simulink model "LOSR"  (R2022a)
settings: Solver=FixedStepDiscrete  StartTime=0.0  StopTime=0.04  FixedStep=0.04  RelTol=1e-3
PreLoadFcn:
  | listing = dir;
  | if (contains([listing .name], 'AGR')) && (contains([listing .name], 'MAP'))
  |     addpath('./AGR', './MAP');
  |     addpath( genpath('./MAP') );
  | elseif (contains([listing .name], 'LOSR.slx'))
  |     addpath('../AGR', '../MAP');
  |     addpath( genpath('../MAP') );
  | else
  | 
  | end
  | 
  | load('BusStructureLOSR.mat');
InitFcn:
  | listing = dir;
  | if (contains([listing .name], 'AGR')) && (contains([listing .name], 'MAP'))
  |     addpath('./AGR', './MAP');
  |     addpath( genpath('./MAP') );
  | elseif (contains([listing .name], 'LOSR.slx'))
  |     addpath('../AGR', '../MAP');
  |     addpath( genpath('../MAP') );
  | else
  | 
  | end
  | 
  | load('BusStructureLOSR.mat');
StartFcn:
  | listing = dir;
  | if (contains([listing .name], 'AGR')) && (contains([listing .name], 'MAP'))
  |     addpath('./AGR', './MAP');
  |     addpath( genpath('./MAP') );
  | elseif (contains([listing .name], 'LOSR.slx'))
  |     addpath('../AGR', '../MAP');
  |     addpath( genpath('../MAP') );
  | else
  | 
  | end
  | 
  | load('BusStructureLOSR.mat');
undefined symbols (not defined in the file or in its folder): b2NED, dCNED, delECEF, isFeasible, llh, losECEF, LOSRDataTagWrap, LOSRDataValid, LOSRDirectionCosineX, LOSRDirectionCosineY, LOSRDirectionCosineZ, LOSRSelected, LOSRSelectedWraparound, LOSRTargetElevation, LOSRTargetLatitude, LOSRTargetLongitude, LOSRTargetRangeEast, LOSRTargetRangeNorth, LOSRTargetRangeVertical, ne, ned2ECEF, pECEF_ref, testLLH, testLLH2, testTerrainHeight
libraries: aerolibconvert2 x2
settings Model: Creator=ASCL  LastModifiedBy=ASCL
settings DataIOCC: SaveOutput=off  SignalLogging=off  DSMLogging=off  SaveTime=off  ReturnWorkspaceOutputs=off
settings OptimizationCC: BlockReduction=off  DefaultParameterBehavior=Inlined  UseDivisionForNetSlopeComputation=on  GainParamInheritBuiltInType=on  UseFloatMulNetSlope=on  ExpressionFolding=off  PassReuseOutputArgsAs=Individual arguments  ZeroExternalMemoryAtStartup=off  ZeroInternalMemoryAtStartup=off  EfficientFloat2IntCast=on  LifeSpan=inf  OptimizeBlockOrder=speed  DifferentSizesBufferReuse=on  EfficientTunableParamExpr=on
settings DebuggingCC: SignalInfNanChecking=warning  ReadBeforeWriteMsg=EnableAllAsWarning  WriteAfterWriteMsg=EnableAllAsError  WriteAfterReadMsg=EnableAllAsError  IntegerOverflowMsg=error  ParameterTunabilityLossMsg=error  UniqueDataStoreMsg=error  AssertControl=DisableAll  NonBusSignalsTreatedAsBus=error  SFInvalidInputDataAccessInChartInitDiag=error  SFTransitionOutsideNaturalParentDiag=error  SFUnreachableExecutionPathDiag=error  SFUndirectedBroadcastEventsDiag=error  IntegerSaturationMsg=error
settings HardwareCC: ProdBitPerPointer=32  ProdBitPerSizeT=32  ProdBitPerPtrDiffT=32  ProdLargestAtomicInteger=Long  ProdLargestAtomicFloat=Double  ProdEndianess=BigEndian  ProdWordSize=32  ProdLongLongMode=on  ProdHWDeviceType=Freescale->MPC83xx
settings ModelReferenceCC: ModelReferenceNumInstancesAllowed=Single
settings SFSimCC: SimCustomHeaderCode="#include \"MAP.h\""  SimUserSources=MAP.c  SimUserLibraries=WS2_32.LIB  CompileTimeRecursionLimit=0  EnableRuntimeRecursion=off  MATLABDynamicMemAlloc=off
settings RTWCC: SystemTargetFile=ert.tlc  TemplateMakefile=ert_default_tmf  GenerateReport=on  RTWUseSimCustomCode=on  CustomHeaderCode="#include \"MAP.h\""  CustomSource=MAP.c  CustomLibrary=WS2_32.LIB  BuildConfiguration=Faster Runs  IncludeHyperlinkInReport=on  LaunchReport=on  GenerateTraceInfo=on  GenerateTraceReport=on  GenerateTraceReportSl=on  GenerateTraceReportSf=on  GenerateTraceReportEml=on  GenerateCodeMetricsReport=on
settings CodeAppCC: ForceParamTrailComments=on  IgnoreCustomStorageClasses=off  OperatorAnnotations=on  SimulinkDataObjDesc=on  SFDataObjDesc=on  MATLABFcnDesc=on  InsertBlockDesc=on  StateflowObjectComments=on  MATLABSourceComments=on  EnableCustomComments=on  InlinedPrmAccess=Macros  ReqsInCode=on
settings ERTTargetCC: TargetLangStandard=C99 (ISO)  UtilityFuncGeneration=Shared location  GenerateSampleERTMain=on  IncludeMdlTerminateFcn=off  CombineSignalStateStructs=on  SuppressErrorStatus=on  SupportAbsoluteTime=off  SupportNonFinite=off  SupportComplex=off  SupportVariableSizeSignals=on  ParenthesesLevel=Standards  CastingMode=Standards  GenerateSharedConstants=off  InlinedParameterPlacement=NonHierarchical  ERTCustomFileTemplate=example_file_process.tlc  RateTransitionBlockCode=Function  PreserveIfCondition=on  ConvertIfToSwitch=off  EnableSignedLeftShifts=off  EnableSignedRightShifts=off

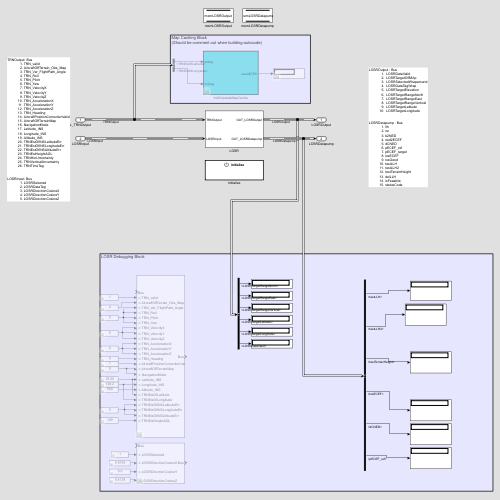
[thumbnail: Simulink's stored preview of the top-level diagram]
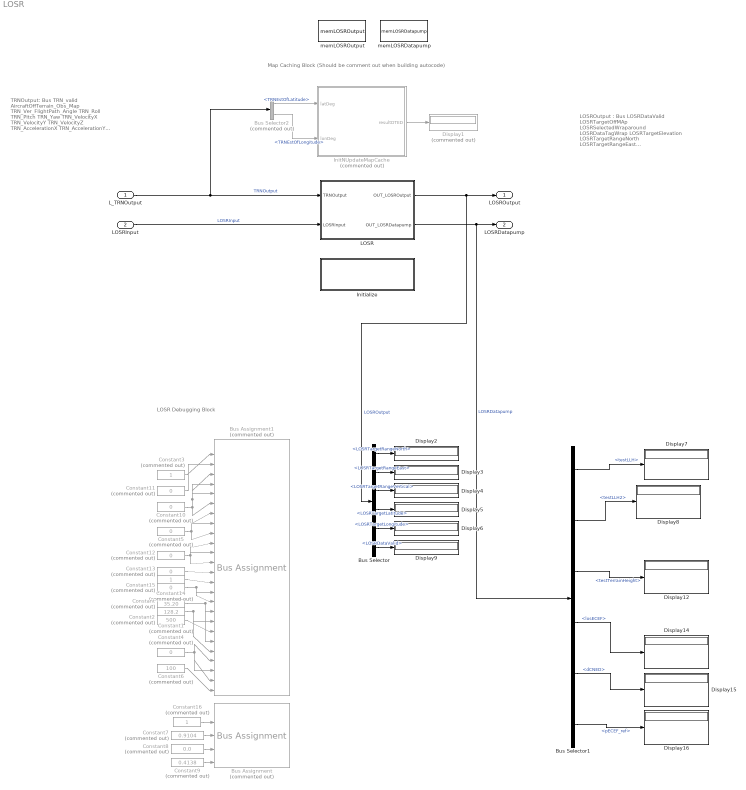
== system LOSR ==
  note: LOSR Debugging Block
  note: LOSROutput : Bus
      | LOSRDataValid
      | LOSRTargetOffMAp
      | LOSRSelectedWraparound
      | LOSRDataTagWrap
      | LOSRTargetElevation
      | LOSRTargetRangeNorth
      | LOSRTargetRangeEast
      | LOSRTargetRangeVertical
      | LOSRTargetLatitude
      | LOSRTargetLongitude
      |
      | LOSRDatapump : Bus
      | llh
      | ne
      | b2NED
      | ned2ECEF
      | dCNED
      | pECEF_ref
      | pECEF_target
      | losECEF
      | losGeod
      | testLLH
      | testLLH2
      | testTerrainHeight
      | delLLH
      | isFeasbile
      | statusCode
  note: TRNOutput: Bus
      | TRN_valid
      | AircraftOffTerrain_Obs_Map
      | TRN_Ver_FlightPath_Angle
      | TRN_Roll
      | TRN_Pitch
      | TRN_Yaw
      | TRN_VelocityX
      | TRN_VelocityY
      | TRN_VelocityZ
      | TRN_AccelerationX
      | TRN_AccelerationY
      | TRN_AccelerationZ
      | TRN_Heading
      | AircraftPositionCorrectionValid
      | AircraftOffTerrainMap
      | NavigationMode
      | Latitude_INS
      | Longitude_INS
      | Altitude_INS
      | TRNEstOfINSLatitudeErr
      | TRNEstOfINSLongitudeErr
      | TRNEstOfINSAltitudeErr
      | TRNEstHeightAGL
      | TRNHorUncertainty
      | TRNVerticalUncertainty
      | TRNTimeTag
      |
      | LOSRInput: Bus
      | LOSRSelected
      | LOSRDataTag
      | LOSRDirectionCosineX
      | LOSRDirectionCosineY
      | LOSRDirectionCosineZ
  note: Map Caching Block
      | (Should be comment out when building autocode)
  L_TRNOutput : Inport  OutDataTypeStr=Bus: TRNOutput  Interpolate=off  BusOutputAsStruct=on
  LOSRInput : Inport  Port=2  OutDataTypeStr=Bus: LOSRInput  Interpolate=off  BusOutputAsStruct=on
  Bus Assignment : BusAssignment  Commented=on  AssignedSignals=LOSRSelected,LOSRDirectionCosineX,LOSRDirectionCosineY,LOSRDirectionCosineZ
  Bus Assignment1 : BusAssignment  Commented=on  AssignedSignals=TRN_valid,AircraftOffTerrain_Obs_Map,TRN_Ver_FlightPath_Angle,TRN_Roll,TRN_Pitch,TRN_Yaw,TRN_VelocityX,TRN_VelocityY,TRN_VelocityZ,TRN_AccelerationX,TRN_AccelerationY,TRN_AccelerationZ,TRN_Heading,AircraftPositionCorrectionValid,AircraftOffTerrainMap,NavigationMode,Latitude_INS,Longitude_INS,Altitude_INS,TRNEstOfLatitude,TRNEstOfLongitude,TRNEstOfINSLatitudeErr,TRNEstOfINSLongitudeErr,TRNEstOfINSAltitudeErr,TRNEstHeightAGL
  Bus Selector : BusSelector  OutputSignals=LOSRTargetRangeNorth,LOSRTargetRangeEast,LOSRTargetRangeVertical,LOSRTargetLatitude,LOSRTargetLongitude,LOSRDataValid
  Bus Selector1 : BusSelector  OutputSignals=testLLH,testLLH2,testTerrainHeight,losECEF,dCNED,pECEF_ref
  Bus Selector2 : BusSelector  Commented=on  OutputSignals=TRNEstOfLatitude,TRNEstOfLongitude
  Constant : Constant  Commented=on  Value=35.20
  Constant1 : Constant  Commented=on  Value=128.2
  Constant{4..5,10,12..13} (5 alike) : Constant  Commented=on  Value=0
  Constant11 : Constant  Commented=on  Value=0  OutDataTypeStr=boolean
  Constant14 : Constant  Commented=on  OutDataTypeStr=boolean
  Constant15 : Constant  Commented=on  Value=0  OutDataTypeStr=boolean
  Constant16 : Constant  Commented=on  OutDataTypeStr=boolean
  Constant2 : Constant  Commented=on  Value=500
  Constant3 : Constant  Commented=on  OutDataTypeStr=boolean
  Constant6 : Constant  Commented=on  Value=100  OutDataTypeStr=uint16
  Constant7 : Constant  Commented=on  Value=0.9104
  Constant8 : Constant  Commented=on  Value=0.0
  Constant9 : Constant  Commented=on  Value=0.4138
  Display1 : Display  Commented=on
  Display{2..9,12,14..16} (12 alike) : Display
  InitNUpdateMapCache : Subsystem  Commented=on  TreatAsAtomicUnit=on
  Initialize : Subsystem  TreatAsAtomicUnit=on
  LOSR : Subsystem
      mask init:
      | % latGPS = double(0);
      | % lonGPS = double(0);
      | % altGPS = double(0);
      | % velEGPS = double(0);
      | % velNGPS = double(0);
      | % velUGPS = double(0);
      | % notValidGPS = boolean(0);
      | % notAvaildINS = boolean(0);
      | % velUINS = double(0);
      | % velVINS = double(0);
      | % velWINS = double(0);
      | % rollINS = double(0);
      | % pitchINS = double(0);
      | % hgdINS = double(0);
      | % accXINS = double(0);
      | % accYINS = double(0);
      | % accZINS = double(0);
      | % activated = boolean(0);
      | % reactionT = uint16(0);
      | % pullUpG = uint16(0);
      | % rollRate = uint16(0);
      | % gOnsetRate = uint16(0);
      | % maxGamma = uint16(0);
      | % setWarnH = double(0);
      | % obsWarningTime = uint16(1);
      | % wiresWarningTime = uint16(1);
      | % latErrOfINS = double(0);
      | % lonErrOfINS = double(0);
      | % altErrorofINS = uint16(0);
      | % heightEstOfTRN = uint16(0);
      | % horUncertaintyOfTRN = double(0);
      | % verUncertaintyOfTRN = double(0);
  memLOSRDatapump : DataStoreMemory  DataStoreName=memLOSRDatapump  ReadBeforeWriteMsg=warning  WriteAfterWriteMsg=warning  WriteAfterReadMsg=warning  VectorParams1D=off  ShowAdditionalParam=off  OutDataTypeStr=Bus: LOSRDatapump
  memLOSROutput : DataStoreMemory  DataStoreName=memLOSROutput  ReadBeforeWriteMsg=warning  WriteAfterWriteMsg=warning  WriteAfterReadMsg=warning  VectorParams1D=off  ShowAdditionalParam=off  OutDataTypeStr=Bus: LOSROutput
  LOSROutput : Outport  OutDataTypeStr=Bus: LOSROutput  VectorParamsAs1DForOutWhenUnconnected=off  BusOutputAsStruct=on
  LOSRDatapump : Outport  Port=2  OutDataTypeStr=Bus: LOSRDatapump  VectorParamsAs1DForOutWhenUnconnected=off  BusOutputAsStruct=on
  wires:
  Constant11/1 -> Bus Assignment1/3
  Constant2/1 -> Bus Assignment1/20
  L_TRNOutput/1 -> Bus Selector2/1, LOSR/1(TRNOutput)  "TRNOutput"
  Constant16/1 -> Bus Assignment/2
  Constant10/1 -> Bus Assignment1/7, Bus Assignment1/4, Bus Assignment1/5, Bus Assignment1/6
  Constant6/1 -> Bus Assignment1/26
  Bus Selector2/2 -> InitNUpdateMapCache/2(lonDeg)  "<TRNEstOfLongitude>"
  Bus Selector/5 -> Display6/1  "<LOSRTargetLongitude>"
  LOSR/2(OUT_LOSRDatapump) -> Bus Selector1/1, LOSRDatapump/1  "LOSRDatapump"
  LOSRInput/1 -> LOSR/2(LOSRInput)  "LOSRInput"
  Constant9/1 -> Bus Assignment/5
  Constant7/1 -> Bus Assignment/3
  Constant1/1 -> Bus Assignment1/22, Bus Assignment1/19
  Bus Selector/2 -> Display3/1  "<LOSRTargetRangeEast>"
  Bus Selector1/2 -> Display8/1  "<testLLH2>"
  Bus Selector1/5 -> Display15/1  "<dCNED>"
  Constant13/1 -> Bus Assignment1/14
  Constant15/1 -> Bus Assignment1/17, Bus Assignment1/16
  Bus Selector/6 -> Display9/1  "<LOSRDataValid>"
  LOSR/1(OUT_LOSROutput) -> Bus Selector/1, LOSROutput/1  "LOSROutput"
  Bus Selector2/1 -> InitNUpdateMapCache/1(latDeg)  "<TRNEstOfLatitude>"
  Constant14/1 -> Bus Assignment1/15
  Bus Selector1/1 -> Display7/1  "<testLLH>"
  Constant12/1 -> Bus Assignment1/13, Bus Assignment1/11, Bus Assignment1/12
  Bus Selector1/6 -> Display16/1  "<pECEF_ref>"
  Constant3/1 -> Bus Assignment1/2
  Constant5/1 -> Bus Assignment1/10, Bus Assignment1/8, Bus Assignment1/9
  Constant4/1 -> Bus Assignment1/23, Bus Assignment1/25, Bus Assignment1/24
  Constant/1 -> Bus Assignment1/21, Bus Assignment1/18
  Bus Selector/4 -> Display5/1  "<LOSRTargetLatitude>"
  Bus Selector/3 -> Display4/1  "<LOSRTargetRangeVertical>"
  Bus Selector/1 -> Display2/1  "<LOSRTargetRangeNorth>"
  Bus Selector1/4 -> Display14/1  "<losECEF>"
  Constant8/1 -> Bus Assignment/4
  Bus Selector1/3 -> Display12/1  "<testTerrainHeight>"
  InitNUpdateMapCache/1(resultDTED) -> Display1/1

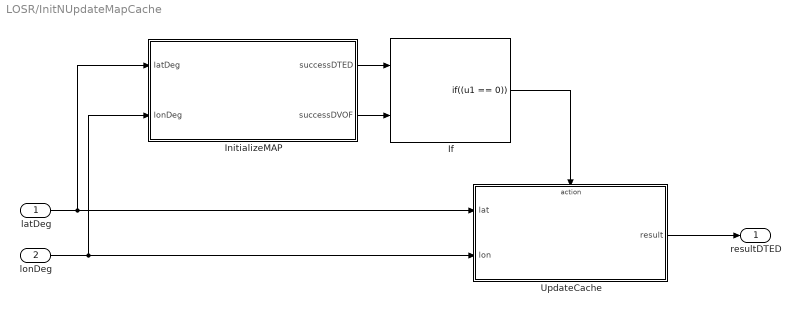
== system LOSR/InitNUpdateMapCache ==
  latDeg : Inport  OutDataTypeStr=double
  lonDeg : Inport  Port=2  OutDataTypeStr=double
  If : If  NumInputs=2  IfExpression=(u1 == 0)  ShowElse=off
  InitializeMAP : MATLAB Function  TreatAsAtomicUnit=on
  UpdateCache : Subsystem  TreatAsAtomicUnit=on
  resultDTED : Outport  VectorParamsAs1DForOutWhenUnconnected=off
  wires:
  lonDeg/1 -> InitializeMAP/2(lonDeg), UpdateCache/2(lon)
  UpdateCache/1(result) -> resultDTED/1
  InitializeMAP/1(successDTED) -> If/1
  latDeg/1 -> InitializeMAP/1(latDeg), UpdateCache/1(lat)
  InitializeMAP/2(successDVOF) -> If/2
  If/1 -> UpdateCache/Action

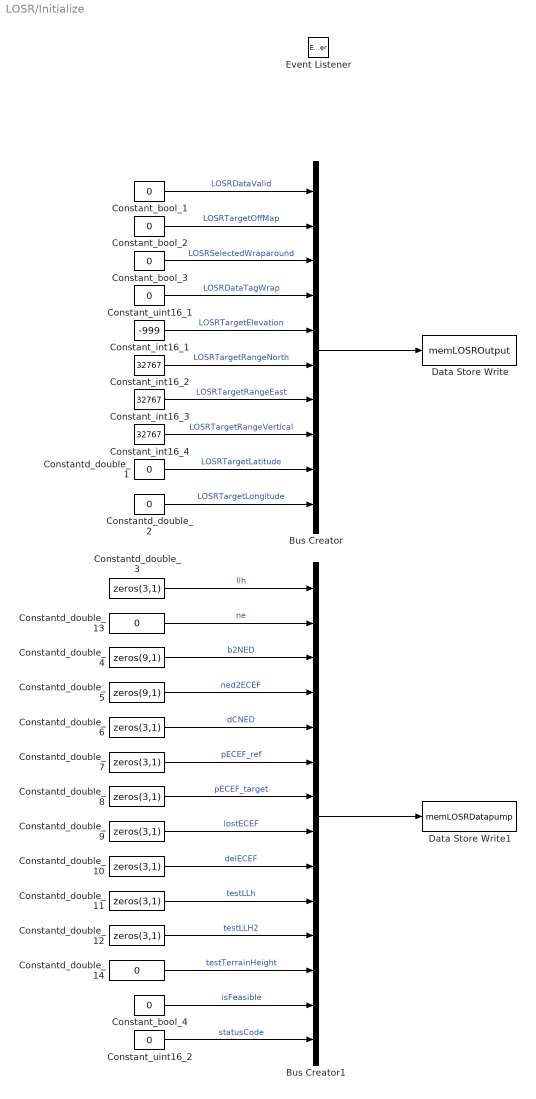
== system LOSR/Initialize ==
  Bus Creator : BusCreator  Inputs=10  OutDataTypeStr=Bus: LOSROutput  NonVirtualBus=on
      settings: InheritFromInputs=off
  Bus Creator1 : BusCreator  Inputs=14  OutDataTypeStr=Bus: LOSRDatapump  NonVirtualBus=on
      settings: InheritFromInputs=off
  Constant_bool_{1..4} (4 alike) : Constant  Value=0  OutDataTypeStr=boolean
  Constant_int16_1 : Constant  Value=-999  OutDataTypeStr=int16
  Constant_int16_2 : Constant  Value=32767  OutDataTypeStr=int16
  Constant_int16_3 : Constant  Value=32767  OutDataTypeStr=int16
  Constant_int16_4 : Constant  Value=32767  OutDataTypeStr=int16
  Constant_uint16_1 : Constant  Value=0  OutDataTypeStr=uint16
  Constant_uint16_2 : Constant  Value=0  OutDataTypeStr=uint16
  Constantd_double_{1..2,13..14} (4 alike) : Constant  Value=0  OutDataTypeStr=double
  Constantd_double_{3,6..12} (8 alike) : Constant  Value=zeros(3,1)  OutDataTypeStr=double
  Constantd_double_4 : Constant  Value=zeros(9,1)  OutDataTypeStr=double
  Constantd_double_5 : Constant  Value=zeros(9,1)  OutDataTypeStr=double
  Data Store Write : DataStoreWrite  DataStoreName=memLOSROutput  IndexOptions=Index vector (dialog)  Indices=1  OutputSizes=1
  Data Store Write1 : DataStoreWrite  DataStoreName=memLOSRDatapump  IndexOptions=Index vector (dialog)  Indices=1  OutputSizes=1
  Event Listener : EventListener  DisableCoverage=on  EventName=reset
  wires:
  Constant_uint16_1/1 -> Bus Creator/4  "LOSRDataTagWrap"
  Constant_bool_1/1 -> Bus Creator/1  "LOSRDataValid"
  Constant_bool_2/1 -> Bus Creator/2  "LOSRTargetOffMap"
  Constant_bool_3/1 -> Bus Creator/3  "LOSRSelectedWraparound"
  Constant_int16_1/1 -> Bus Creator/5  "LOSRTargetElevation"
  Constant_int16_2/1 -> Bus Creator/6  "LOSRTargetRangeNorth"
  Constant_int16_3/1 -> Bus Creator/7  "LOSRTargetRangeEast"
  Constant_int16_4/1 -> Bus Creator/8  "LOSRTargetRangeVertical"
  Constantd_double_1/1 -> Bus Creator/9  "LOSRTargetLatitude"
  Constantd_double_2/1 -> Bus Creator/10  "LOSRTargetLongitude"
  Bus Creator/1 -> Data Store Write/1
  Bus Creator1/1 -> Data Store Write1/1
  Constantd_double_3/1 -> Bus Creator1/1  "llh"
  Constantd_double_4/1 -> Bus Creator1/3  "b2NED"
  Constantd_double_5/1 -> Bus Creator1/4  "ned2ECEF"
  Constantd_double_8/1 -> Bus Creator1/7  "pECEF_target"
  Constantd_double_7/1 -> Bus Creator1/6  "pECEF_ref"
  Constantd_double_6/1 -> Bus Creator1/5  "dCNED"
  Constantd_double_9/1 -> Bus Creator1/8  "lostECEF"
  Constantd_double_10/1 -> Bus Creator1/9  "delECEF"
  Constantd_double_11/1 -> Bus Creator1/10  "testLLh"
  Constantd_double_12/1 -> Bus Creator1/11  "testLLH2"
  Constantd_double_13/1 -> Bus Creator1/2  "ne"
  Constantd_double_14/1 -> Bus Creator1/12  "testTerrainHeight"
  Constant_bool_4/1 -> Bus Creator1/13  "isFeasible"
  Constant_uint16_2/1 -> Bus Creator1/14  "statusCode"

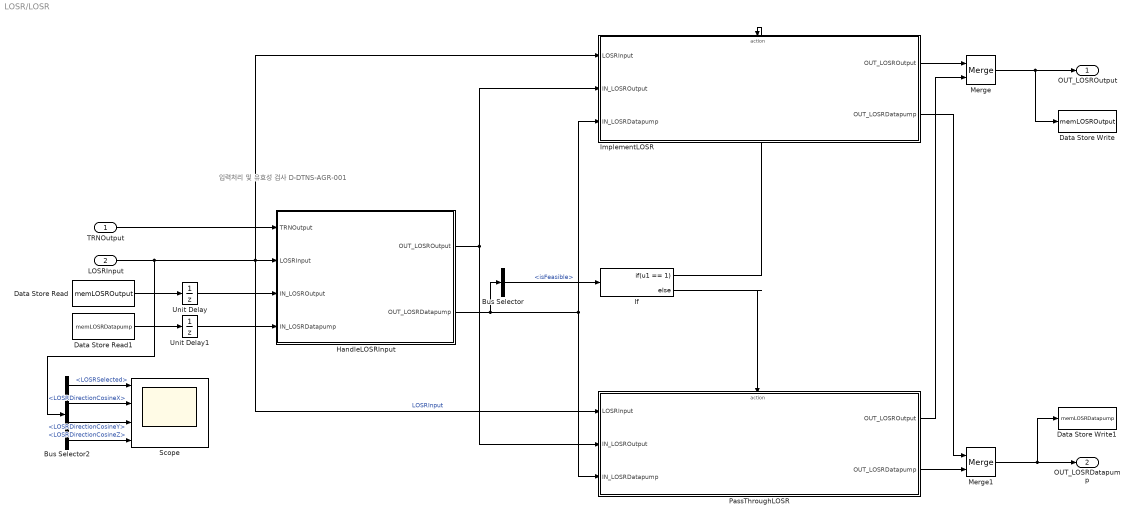
== system LOSR/LOSR ==
  note: 입력처리 및 유효성 검사 D-DTNS-AGR-001
  TRNOutput : Inport  OutDataTypeStr=Bus: TRNOutput
  LOSRInput : Inport  Port=2  OutDataTypeStr=Bus: LOSRInput
  Bus Selector : BusSelector  OutputSignals=isFeasible
  Bus Selector2 : BusSelector  OutputSignals=LOSRSelected,LOSRDirectionCosineX,LOSRDirectionCosineY,LOSRDirectionCosineZ
  Data Store Read : DataStoreRead  DataStoreName=memLOSROutput  IndexOptions=Index vector (dialog)  Indices=1  OutputSizes=1
  Data Store Read1 : DataStoreRead  DataStoreName=memLOSRDatapump  IndexOptions=Index vector (dialog)  Indices=1  OutputSizes=1
  Data Store Write : DataStoreWrite  DataStoreName=memLOSROutput  IndexOptions=Index vector (dialog)  Indices=1  OutputSizes=1
  Data Store Write1 : DataStoreWrite  DataStoreName=memLOSRDatapump  IndexOptions=Index vector (dialog)  Indices=1  OutputSizes=1
  HandleLOSRInput : Subsystem  TreatAsAtomicUnit=on
      settings: RTWSystemCode=Nonreusable function  RTWFcnNameOpts=Use subsystem name
  If : If  IfExpression=u1 == 1
  ImplementLOSR : Subsystem  TreatAsAtomicUnit=on
      settings: RTWSystemCode=Nonreusable function  RTWFcnNameOpts=Use subsystem name
  Merge : Merge
  Merge1 : Merge
  PassThroughLOSR : Subsystem  TreatAsAtomicUnit=on
      settings: RTWSystemCode=Nonreusable function  RTWFcnNameOpts=Use subsystem name
  Scope : Scope  NumInputPorts=4
  Unit Delay : UnitDelay  SampleTime=-1  HasFrameUpgradeWarning=on
  Unit Delay1 : UnitDelay  SampleTime=-1  HasFrameUpgradeWarning=on
  OUT_LOSROutput : Outport  OutDataTypeStr=Bus: LOSROutput  VectorParamsAs1DForOutWhenUnconnected=off
  OUT_LOSRDatapump : Outport  Port=2  OutDataTypeStr=Bus: LOSRDatapump  VectorParamsAs1DForOutWhenUnconnected=off
  wires:
  LOSRInput/1 -> Bus Selector2/1, ImplementLOSR/1(LOSRInput), PassThroughLOSR/1(LOSRInput), HandleLOSRInput/2(LOSRInput)  "LOSRInput"
  HandleLOSRInput/1(OUT_LOSROutput) -> PassThroughLOSR/2(IN_LOSROutput), ImplementLOSR/2(IN_LOSROutput)
  Bus Selector/1 -> If/1  "<isFeasible>"
  If/1 -> ImplementLOSR/Action
  HandleLOSRInput/2(OUT_LOSRDatapump) -> Bus Selector/1, ImplementLOSR/3(IN_LOSRDatapump), PassThroughLOSR/3(IN_LOSRDatapump)
  ImplementLOSR/1(OUT_LOSROutput) -> Merge/1
  PassThroughLOSR/2(OUT_LOSRDatapump) -> Merge1/2
  ImplementLOSR/2(OUT_LOSRDatapump) -> Merge1/1
  PassThroughLOSR/1(OUT_LOSROutput) -> Merge/2
  Merge/1 -> Data Store Write/1, OUT_LOSROutput/1
  Merge1/1 -> Data Store Write1/1, OUT_LOSRDatapump/1
  If/2 -> PassThroughLOSR/Action
  TRNOutput/1 -> HandleLOSRInput/1(TRNOutput)
  Data Store Read/1 -> Unit Delay/1
  Data Store Read1/1 -> Unit Delay1/1
  Unit Delay/1 -> HandleLOSRInput/3(IN_LOSROutput)
  Unit Delay1/1 -> HandleLOSRInput/4(IN_LOSRDatapump)
  Bus Selector2/1 -> Scope/1  "<LOSRSelected>"
  Bus Selector2/2 -> Scope/2  "<LOSRDirectionCosineX>"
  Bus Selector2/3 -> Scope/3  "<LOSRDirectionCosineY>"
  Bus Selector2/4 -> Scope/4  "<LOSRDirectionCosineZ>"

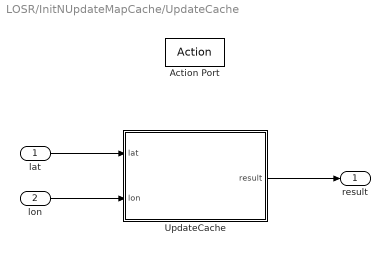
== system LOSR/InitNUpdateMapCache/UpdateCache ==
  lat : Inport
  lon : Inport  Port=2
  Action Port : ActionPort
  UpdateCache : MATLAB Function  TreatAsAtomicUnit=on
  result : Outport  VectorParamsAs1DForOutWhenUnconnected=off
  wires:
  UpdateCache/1(result) -> result/1
  lat/1 -> UpdateCache/1(lat)
  lon/1 -> UpdateCache/2(lon)

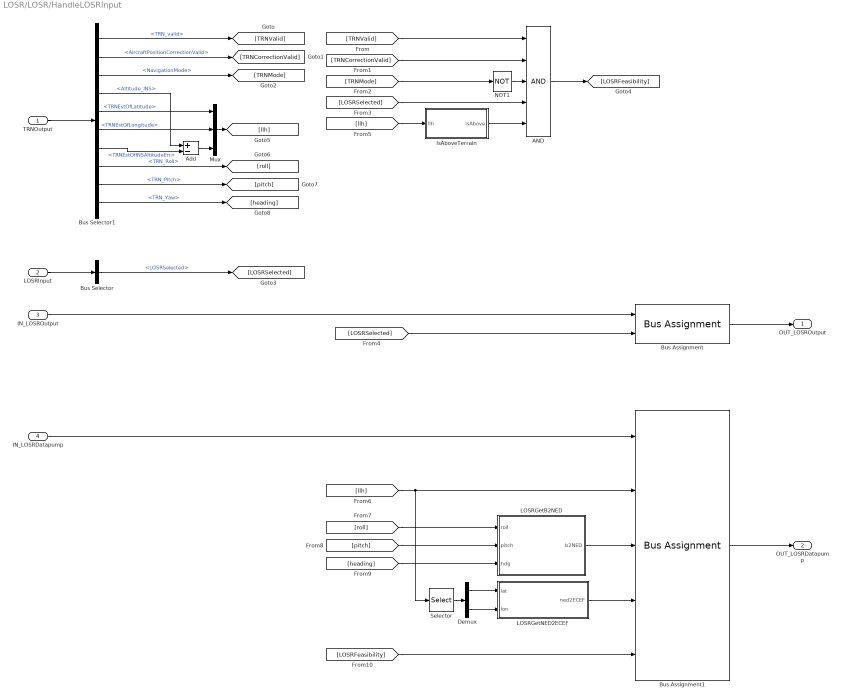
== system LOSR/LOSR/HandleLOSRInput ==
  TRNOutput : Inport  OutDataTypeStr=Bus: TRNOutput
  LOSRInput : Inport  Port=2  OutDataTypeStr=Bus: LOSRInput
  IN_LOSROutput : Inport  Port=3  OutDataTypeStr=Bus: LOSROutput
  IN_LOSRDatapump : Inport  Port=4  OutDataTypeStr=Bus: LOSRDatapump
  AND : Logic  Inputs=5  AllPortsSameDT=off  OutDataTypeStr=boolean
  Add : Sum  Inputs=+-
  Bus Assignment : BusAssignment  AssignedSignals=LOSRSelectedWraparound
  Bus Assignment1 : BusAssignment  AssignedSignals=llh,b2NED,ned2ECEF,isFeasible
  Bus Selector : BusSelector  OutputSignals=LOSRSelected
  Bus Selector1 : BusSelector  OutputSignals=TRN_valid,AircraftPositionCorrectionValid,NavigationMode,Altitude_INS,TRNEstOfLatitude,TRNEstOfLongitude,TRNEstOfINSAltitudeErr,TRN_Roll,TRN_Pitch,TRN_Yaw
  Demux : Demux  Outputs=2
  IsAboveTerrain : MATLAB Function  TreatAsAtomicUnit=on
  LOSRGetB2NED : MATLAB Function  TreatAsAtomicUnit=on
  LOSRGetNED2ECEF : MATLAB Function  TreatAsAtomicUnit=on
  Mux : Mux  Inputs=3
  NOT1 : Logic  Operator=NOT  IconShape=distinctive  AllPortsSameDT=off  OutDataTypeStr=boolean
  Selector : Selector  InputPortWidth=3  IndexOptions=Index vector (dialog)  Indices=[1 2]  OutputSizes=1
  OUT_LOSROutput : Outport  OutDataTypeStr=Bus: LOSROutput  VectorParamsAs1DForOutWhenUnconnected=off
  OUT_LOSRDatapump : Outport  Port=2  OutDataTypeStr=Bus: LOSRDatapump  VectorParamsAs1DForOutWhenUnconnected=off
  wires:
  IN_LOSRDatapump/1 -> Bus Assignment1/1
  IN_LOSROutput/1 -> Bus Assignment/1
  TRNOutput/1 -> Bus Selector1/1
  Bus Selector1/1 -> [TRNValid]  "<TRN_valid>"
  Bus Selector1/2 -> [TRNCorrectionValid]  "<AircraftPositionCorrectionValid>"
  Bus Selector1/3 -> [TRNMode]  "<NavigationMode>"
  LOSRInput/1 -> Bus Selector/1
  Bus Selector/1 -> [LOSRSelected]  "<LOSRSelected>"
  [TRNValid] -> AND/1
  [TRNCorrectionValid] -> AND/2
  [TRNMode] -> NOT1/1
  [LOSRSelected] -> AND/4
  AND/1 -> [LOSRFeasibility]
  Bus Assignment1/1 -> OUT_LOSRDatapump/1
  LOSRGetNED2ECEF/1(ned2ECEF) -> Bus Assignment1/4
  LOSRGetB2NED/1(b2NED) -> Bus Assignment1/3
  Bus Selector1/4 -> Add/1  "<Altitude_INS>"
  Bus Selector1/5 -> Mux/1  "<TRNEstOfLatitude>"
  Bus Selector1/6 -> Mux/2  "<TRNEstOfLongitude>"
  Add/1 -> Mux/3
  Bus Selector1/7 -> Add/2  "<TRNEstOfINSAltitudeErr>"
  Mux/1 -> [llh]
  Bus Selector1/10 -> [heading]  "<TRN_Yaw>"
  Bus Selector1/9 -> [pitch]  "<TRN_Pitch>"
  Bus Selector1/8 -> [roll]  "<TRN_Roll>"
  [llh] -> Selector/1, Bus Assignment1/2
  Selector/1 -> Demux/1
  Demux/2 -> LOSRGetNED2ECEF/2(lon)
  Demux/1 -> LOSRGetNED2ECEF/1(lat)
  [roll] -> LOSRGetB2NED/1(roll)
  [pitch] -> LOSRGetB2NED/2(pitch)
  [heading] -> LOSRGetB2NED/3(hdg)
  NOT1/1 -> AND/3
  [LOSRFeasibility] -> Bus Assignment1/5
  Bus Assignment/1 -> OUT_LOSROutput/1
  [LOSRSelected] -> Bus Assignment/2
  [llh] -> IsAboveTerrain/1(llh)
  IsAboveTerrain/1(isAbove) -> AND/5

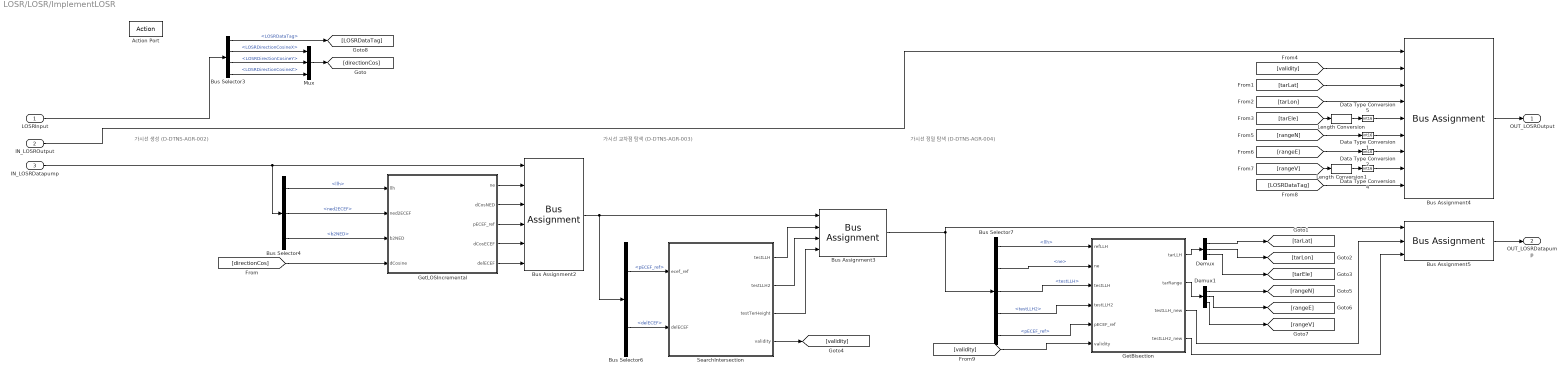
== system LOSR/LOSR/ImplementLOSR ==
  note: 가시선 생성 (D-DTNS-AGR-002)
  note: 가시선 교차점 탐색 (D-DTNS-AGR-003)
  note: 가시선 정밀 탐색 (D-DTNS-AGR-004)
  LOSRInput : Inport  OutDataTypeStr=Bus: LOSRInput
  IN_LOSROutput : Inport  Port=2  OutDataTypeStr=Bus: LOSROutput
  IN_LOSRDatapump : Inport  Port=3  OutDataTypeStr=Bus: LOSRDatapump
  Action Port : ActionPort  ActionPortLabel=if(u1 == 1)
  Bus Assignment2 : BusAssignment  AssignedSignals=ne,dCNED,pECEF_ref,losECEF,delECEF
  Bus Assignment3 : BusAssignment  AssignedSignals=testLLH,testLLH2,testTerrainHeight
  Bus Assignment4 : BusAssignment  AssignedSignals=LOSRDataValid,LOSRTargetLatitude,LOSRTargetLongitude,LOSRTargetElevation,LOSRTargetRangeNorth,LOSRTargetRangeEast,LOSRTargetRangeVertical,LOSRDataTagWrap
  Bus Assignment5 : BusAssignment  AssignedSignals=testLLH,testLLH2
  Bus Selector3 : BusSelector  OutputSignals=LOSRDataTag,LOSRDirectionCosineX,LOSRDirectionCosineY,LOSRDirectionCosineZ
  Bus Selector4 : BusSelector  OutputSignals=llh,ned2ECEF,b2NED
  Bus Selector6 : BusSelector  OutputSignals=pECEF_ref,delECEF
  Bus Selector7 : BusSelector  OutputSignals=llh,ne,testLLH,testLLH2,pECEF_ref
  Data Type Conversion{1..2,4..5} (4 alike) : DataTypeConversion  OutDataTypeStr=int16  RndMeth=Floor
  Demux : Demux  Outputs=3
  Demux1 : Demux  Outputs=3
  GetBisection : MATLAB Function  TreatAsAtomicUnit=on
      settings: RTWSystemCode=Nonreusable function  RTWFcnNameOpts=Use subsystem name
  GetLOSIncremental : MATLAB Function  TreatAsAtomicUnit=on
      settings: RTWSystemCode=Nonreusable function  RTWFcnNameOpts=Use subsystem name
  Length Conversion : aerolibconvert2/Length Conversion  IU=m  OU=ft
  Length Conversion1 : aerolibconvert2/Length Conversion  IU=m  OU=ft
  Mux : Mux  Inputs=3
  SearchIntersection : MATLAB Function  TreatAsAtomicUnit=on
      settings: RTWSystemCode=Nonreusable function  RTWFcnNameOpts=Use subsystem name
  OUT_LOSROutput : Outport  OutDataTypeStr=Bus: LOSROutput  VectorParamsAs1DForOutWhenUnconnected=off
  OUT_LOSRDatapump : Outport  Port=2  OutDataTypeStr=Bus: LOSRDatapump  VectorParamsAs1DForOutWhenUnconnected=off
  wires:
  Bus Assignment3/1 -> Bus Selector7/1, Bus Assignment5/1
  SearchIntersection/4(validity) -> [validity]
  [tarLat] -> Bus Assignment4/3
  SearchIntersection/1(testLLH) -> Bus Assignment3/2
  [rangeV] -> Length Conversion1/1
  [directionCos] -> GetLOSIncremental/4(dCosine)
  [tarEle] -> Length Conversion/1
  Bus Selector4/3 -> GetLOSIncremental/3(b2NED)  "<b2NED>"
  Bus Assignment2/1 -> Bus Selector6/1, Bus Assignment3/1
  [tarLon] -> Bus Assignment4/4
  Bus Selector3/3 -> Mux/2  "<LOSRDirectionCosineY>"
  Bus Selector3/2 -> Mux/1  "<LOSRDirectionCosineX>"
  IN_LOSRDatapump/1 -> Bus Selector4/1, Bus Assignment2/1
  Bus Selector4/1 -> GetLOSIncremental/1(llh)  "<llh>"
  Bus Selector3/1 -> [LOSRDataTag]  "<LOSRDataTag>"
  Bus Selector4/2 -> GetLOSIncremental/2(ned2ECEF)  "<ned2ECEF>"
  IN_LOSROutput/1 -> Bus Assignment4/1
  [rangeN] -> Data Type Conversion1/1
  Demux1/2 -> [rangeE]
  Demux1/1 -> [rangeN]
  Mux/1 -> [directionCos]
  [rangeE] -> Data Type Conversion2/1
  Demux/3 -> [tarEle]
  SearchIntersection/3(testTerHeight) -> Bus Assignment3/4
  Demux1/3 -> [rangeV]
  [validity] -> Bus Assignment4/2
  LOSRInput/1 -> Bus Selector3/1
  Bus Assignment4/1 -> OUT_LOSROutput/1
  Bus Assignment5/1 -> OUT_LOSRDatapump/1
  Bus Selector3/4 -> Mux/3  "<LOSRDirectionCosineZ>"
  [LOSRDataTag] -> Bus Assignment4/9
  GetLOSIncremental/5(delECEF) -> Bus Assignment2/6
  GetLOSIncremental/1(ne) -> Bus Assignment2/2
  GetLOSIncremental/2(dCosNED) -> Bus Assignment2/3
  GetLOSIncremental/3(pECEF_ref) -> Bus Assignment2/4
  GetLOSIncremental/4(dCosECEF) -> Bus Assignment2/5
  Bus Selector6/1 -> SearchIntersection/1(ecef_ref)  "<pECEF_ref>"
  Bus Selector6/2 -> SearchIntersection/2(delECEF)  "<delECEF>"
  SearchIntersection/2(testLLH2) -> Bus Assignment3/3
  Bus Selector7/1 -> GetBisection/1(refLLH)  "<llh>"
  Bus Selector7/2 -> GetBisection/2(ne)  "<ne>"
  Bus Selector7/3 -> GetBisection/3(testLLH)  "<testLLH>"
  Bus Selector7/4 -> GetBisection/4(testLLH2)  "<testLLH2>"
  Bus Selector7/5 -> GetBisection/5(pECEF_ref)  "<pECEF_ref>"
  GetBisection/1(tarLLH) -> Demux/1
  Demux/1 -> [tarLat]
  Demux/2 -> [tarLon]
  GetBisection/2(tarRange) -> Demux1/1
  GetBisection/4(testLLH2_new) -> Bus Assignment5/3
  GetBisection/3(testLLH_new) -> Bus Assignment5/2
  [validity] -> GetBisection/6(validity)
  Length Conversion/1 -> Data Type Conversion5/1
  Data Type Conversion4/1 -> Bus Assignment4/8
  Data Type Conversion5/1 -> Bus Assignment4/5
  Length Conversion1/1 -> Data Type Conversion4/1
  Data Type Conversion1/1 -> Bus Assignment4/6
  Data Type Conversion2/1 -> Bus Assignment4/7

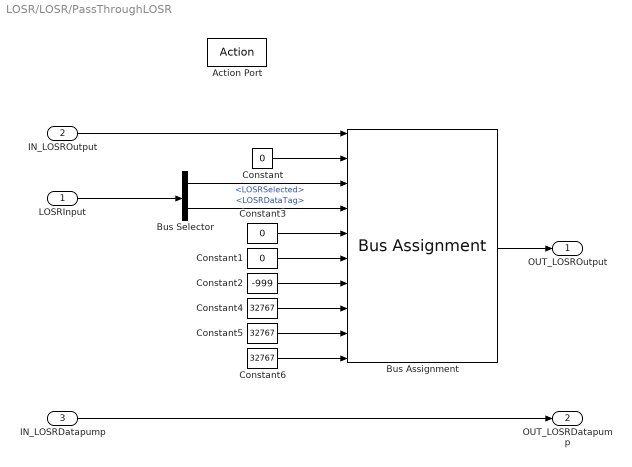
== system LOSR/LOSR/PassThroughLOSR ==
  LOSRInput : Inport  OutDataTypeStr=Bus: LOSRInput
  IN_LOSROutput : Inport  Port=2  OutDataTypeStr=Bus: LOSROutput
  IN_LOSRDatapump : Inport  Port=3  OutDataTypeStr=Bus: LOSRDatapump
  Action Port : ActionPort  ActionPortLabel=else
  Bus Assignment : BusAssignment  AssignedSignals=LOSRDataValid,LOSRSelectedWraparound,LOSRDataTagWrap,LOSRTargetLatitude,LOSRTargetLongitude,LOSRTargetElevation,LOSRTargetRangeNorth,LOSRTargetRangeEast,LOSRTargetRangeVertical
  Bus Selector : BusSelector  OutputSignals=LOSRSelected,LOSRDataTag
  Constant : Constant  Value=0  OutDataTypeStr=boolean
  Constant1 : Constant  Value=0
  Constant2 : Constant  Value=-999  OutDataTypeStr=int16
  Constant3 : Constant  Value=0
  Constant4 : Constant  Value=32767  OutDataTypeStr=int16
  Constant5 : Constant  Value=32767  OutDataTypeStr=int16
  Constant6 : Constant  Value=32767  OutDataTypeStr=int16
  OUT_LOSROutput : Outport  OutDataTypeStr=Bus: LOSROutput  VectorParamsAs1DForOutWhenUnconnected=off
  OUT_LOSRDatapump : Outport  Port=2  OutDataTypeStr=Bus: LOSRDatapump  VectorParamsAs1DForOutWhenUnconnected=off
  wires:
  IN_LOSROutput/1 -> Bus Assignment/1
  IN_LOSRDatapump/1 -> OUT_LOSRDatapump/1
  LOSRInput/1 -> Bus Selector/1
  Constant/1 -> Bus Assignment/2
  Bus Assignment/1 -> OUT_LOSROutput/1
  Bus Selector/1 -> Bus Assignment/3  "<LOSRSelected>"
  Bus Selector/2 -> Bus Assignment/4  "<LOSRDataTag>"
  Constant1/1 -> Bus Assignment/6
  Constant3/1 -> Bus Assignment/5
  Constant4/1 -> Bus Assignment/8
  Constant5/1 -> Bus Assignment/9
  Constant6/1 -> Bus Assignment/10
  Constant2/1 -> Bus Assignment/7

== matlab function LOSR/InitNUpdateMapCache/UpdateCache/UpdateCache ==
  data: result output; lat input; lon input
function result = UpdateCache(lat, lon)
%UpdateCache

% Persistent variables
persistent latPrev lonPrev
if isempty(latPrev)
    latPrev = 0.0;
end
if isempty(lonPrev)
    lonPrev = 0.0;
end

% Initialize output
result = int32(1);

if ( abs(lat - latPrev) > 0.05 ) || ( abs(lon - lonPrev) > 0.05)
    result = coder.ceval('UpdateCache', lat, lon);
    latPrev = lat;
    lonPrev = lon;
else
    
end

== matlab function LOSR/InitNUpdateMapCache/InitializeMAP ==
  data: successDTED output; successDVOF output; latDeg input; lonDeg input
function [successDTED, successDVOF] = InitializeMAP(latDeg, lonDeg)
%InitializeMAP

% Persistent variable
persistent firstRun
if isempty(firstRun)
    firstRun = true;
end

% Initialize output
flagDTED = int32(1);
flagDVOF = int32(1);
successDTED = int32(1);
successDVOF = int32(1);
hDEM = 0.0;

if firstRun
    % Path of DTED data
    pathDTED = 'C:\Users\ASCL\Documents\GitHub\DTNS\MAP\MAP_DB';

    % Length of DETD data path
    strLenDTED = int32(strlength(pathDTED));
    
    hDEM = coder.ceval('MAPGetTerrainHeight', latDeg, lonDeg);
    if IsNear(hDEM, -1.0)
        % Call [ InitialMap ] : 맵 폴더 위치 설정
        flagDTED = coder.ceval('InitialMap', pathDTED, strLenDTED );
        successDTED = flagDTED;
        if (~successDTED)
            firstRun = false;
        end
    else
        successDTED = int32(0);
        firstRun = false;       
    end
else
    successDTED = int32(0);
    successDVOF = int32(0);
end

== matlab function LOSR/HandleLOSRInput/IsAboveTerrain ==
  data: llh input; isAbove output
function isAbove = IsAboveTerrain(llh)
%IsAboveTerrain 현재 항공기 고도가 지형고도 보다 위에 있는지 확인

isAbove = true;
hDEM = 0.0;

hDEM = coder.ceval('MAPGetTerrainHeight', llh(1), llh(2));

if (llh(3) > hDEM)
    isAbove = true;
else
    isAbove = false;
end

== matlab function LOSR/ImplementLOSR/GetLOSIncremental ==
  data: ne output; dCosNED output; pECEF_ref output; dCosECEF output; delECEF output; llh input; ned2ECEF input; b2NED input; dCosine input
function [ne, dCosNED, pECEF_ref, dCosECEF, delECEF] = GetLOSIncremental(llh, ned2ECEF, b2NED, dCosine)
%GetLOSIncremental
% Compute Direction Cosine in NED frame using Body to NED transformation
% Input
% llh       : Current aircraft latitude[deg], longitude[deg], altitude[m]
% b2NED     : Body to NED Transformation Matrix
% dCosine   : Direction Cosine X, Y, Z
% Output
% delLLH
% pECEF_ref
% losECEF
% losGeod
% ne        : Prime vertical radius of curvature

% Initialize Output
dCosNED         = zeros(3,1);
pECEF_ref       = zeros(3,1);
dCosECEF        = zeros(3,1);
delECEF         = zeros(3,1);

% Arrange inputs & internal variables
lat             = llh(1);
lon             = llh(2);
alt             = llh(3);

% Define constants
R_Ea            = 6378137.0;        % Earth semi-major axis [m]
e               = 0.08181919;       % Earth eccentricity
% LOSI_MAX_RANGE  = 28290.0;
% LOSI_MAX_STEPS  = 944;
LOSI_STEP_SIZE  = 30.0;

% Prime vertical radius of curvature
ne              = R_Ea / sqrt(1 - (e * sind(lat))^2 );

% Define reference point in ECEF coordinates
pECEF_ref(1)    = (ne+alt) * cosd(lat) * cosd(lon);
pECEF_ref(2)    = (ne+alt) * cosd(lat) * sind(lon);
pECEF_ref(3)    = (ne * ( 1 - e^2 ) + alt) * sind(lat);

% Direction Cosine in NED
dCosNED(1) = b2NED(1)*dCosine(1) + b2NED(2)*dCosine(2) + b2NED(3)*dCosine(3);
dCosNED(2) = b2NED(4)*dCosine(1) + b2NED(5)*dCosine(2) + b2NED(6)*dCosine(3);
dCosNED(3) = b2NED(7)*dCosine(1) + b2NED(8)*dCosine(2) + b2NED(9)*dCosine(3);

% Direction Cosine in ECEF
dCosECEF(1) = ...
    ned2ECEF(1)*dCosNED(1) +ned2ECEF(2)*dCosNED(2) +ned2ECEF(3)*dCosNED(3);
dCosECEF(2) = ...
    ned2ECEF(4)*dCosNED(1) +ned2ECEF(5)*dCosNED(2) +ned2ECEF(6)*dCosNED(3);
dCosECEF(3) = ...
    ned2ECEF(7)*dCosNED(1) +ned2ECEF(8)*dCosNED(2) +ned2ECEF(9)*dCosNED(3);

% LOS serach vector in ECEF
delECEF = LOSI_STEP_SIZE * dCosECEF;

end

== matlab function LOSR/ImplementLOSR/SearchIntersection ==
  data: ecef_ref input; delECEF input; testLLH output; testLLH2 output; testTerHeight output; validity output
function [testLLH, testLLH2, testTerHeight, validity] = SearchIntersection(ecef_ref, delECEF)

% Initialize Variables
testLLH         = zeros(3,1);
testLLH2        = zeros(3,1);
testECEF        = zeros(3,1);
testTerHeight   = 0.0;
validity        = true;

% Define
% LOSI_MAX_RANGE  = 28290.0;
LOSI_MAX_STEPS  = 944;
% LOSI_STEP_SIZE  = 30.0;

% Searching LOS Intersection
for ii=0:(LOSI_MAX_STEPS-1)
    testECEF(1) = ecef_ref(1) + ii*delECEF(1);
    testECEF(2) = ecef_ref(2) + ii*delECEF(2);
    testECEF(3) = ecef_ref(3) + ii*delECEF(3);
    
    testLLH2    = testLLH;
    testLLH     = ConvertECEF2LLH(testECEF);

    % Get Terrain Elevation
    testTerHeight  = coder.ceval('MAPGetTerrainHeight', testLLH(1), testLLH(2));
    
    if (testTerHeight >= testLLH(3))
        % Itersection found
        if ii==0
            % LOS Intersection is not possible
            validity = false;
            testLLH2 = testLLH;
            break;
        else
            % LOS Intersection exists
            validity = true;
            break;
        end
        
    else
        % Intersection not found yet
        if (ii==(LOSI_MAX_STEPS-1))
        % Max iteration is over without intersection found
        validity = false;
        end
        continue;
    end
    
end

end

function llh  = ConvertECEF2LLH(xyzECEF)
%ConvertECEF2LLH
% Compute the {LLH} coordinates given {ECEF} coordinates
%
% == Inputs =========
% ecef              -  {ECEF} coordinates [m, m, m]
%
% == Outputs ========
% llh               - Corresponding Latitude, Longitude, Height [deg,deg,m]
%

% Initialize
llh = zeros(3,1);
lat     = 0.0;
lon     = 0.0;
h       = 0.0;

% WGS84 Parameters
r_e     = 6378137.0;            % major
f       = 1/298.257223563;      % (first) flattening
r_b     = r_e * (1-f);          % minor
e       = 0.08181919;           % Earth eccentricity
e2      = e*e;                  % Square of Earth eccentricity

% Rearrange
x       = xyzECEF(1);
y       = xyzECEF(2);
z       = xyzECEF(3);

% Longitude
lon = atan2d(y, x);

% Iteration for Latitude and Height [Bowring's method]

% Iteration parameters
eps     = 1;
tol     = 1e-12;

% side of triagle (hypotenuse: N+h, other side: z+N*e2*sind(lat) )
s       = sqrt(x^2 + y^2);

% Initial guesses
h   = 0.0;
N   = r_e;
lat = atand( z / (s * (1-e2*N/(N+h))) );

% Iteration terminates within 3~4 iterations.
count   = 0;

while (eps > tol) || (count > 10)
    lat0 = lat;

    % Recalculate
    h = s / cosd(lat) - N; 
    N   = r_e / sqrt(1-e2*(sind(lat))^2);
    lat = atand( z / (s * (1-e2*N/(N+h))) );

    % Update terminal condition parameters
    eps = abs(lat - lat0);
    count = count + 1;
end

llh = [lat; lon; h];

end

== matlab function LOSR/ImplementLOSR/GetBisection ==
  data: refLLH input; ne input; testLLH input; testLLH2 input; tarLLH output; tarRange output; testLLH_new output; pECEF_ref input; testLLH2_new output; validity input
function [tarLLH, tarRange, testLLH_new, testLLH2_new]   = GetBisection(refLLH, ne, testLLH, testLLH2, pECEF_ref, validity)
%GetBisection
% Initialize Output
tarLLH      = zeros(3,1);
tarRange    = zeros(3,1);
testLLH_new = zeros(3,1);
testLLH2_new= zeros(3,1);

pECEF_target= zeros(3,1);
ecef2NED    = zeros(3,3);
testTerHeight = 0.0;

% Constants
MAX_BISECTION   = 30;
TOL_BISECTION   = 0.5;

if (validity == false)
    tarLLH      = zeros(3,1);
    tarLLH(3)   = -304.495;
    tarRange = [32767; 32767; 9987.3816];
    
else
    for ii=0:(MAX_BISECTION -1)
        testTerHeight = coder.ceval('MAPGetTerrainHeight', (testLLH(1) + testLLH2(1))/2, (testLLH(2) + testLLH2(2))/2 );

        if ( abs(testTerHeight - (testLLH(3)+testLLH2(3))/2) < TOL_BISECTION )
            break;
        end

        if ( testTerHeight < (testLLH(3) + testLLH2(3))/2 )
            testLLH2(1)     = (testLLH(1) + testLLH2(1)) /2;
            testLLH2(2)     = (testLLH(2) + testLLH2(2)) /2;
            testLLH2(3)     = (testLLH(3) + testLLH2(3)) /2;
        else
            testLLH(1)      = (testLLH(1) + testLLH2(1)) /2;
            testLLH(2)      = (testLLH(2) + testLLH2(2)) /2;
            testLLH(3)      = (testLLH(3) + testLLH2(3)) /2;
        end

    end
    
    EARTH_ECCENTRICITY      = 0.08181919;
    
    testLLH_new         = testLLH;
    testLLH2_new        = testLLH2;
    tarLLH              = (testLLH + testLLH2) /2;
    
    % Calculate Output
    pECEF_target(1)     = (ne + testTerHeight)*cosd(tarLLH(1))*cosd(tarLLH(2));
    pECEF_target(2)     = (ne + testTerHeight)*cosd(tarLLH(1))*sind(tarLLH(2));
    pECEF_target(3)     = (ne * (1 - EARTH_ECCENTRICITY^2) + testTerHeight) * sind(tarLLH(1));

    ecef2NED    = [ -sind(refLLH(1)) * cosd(refLLH(2)), -sind(refLLH(1)) * sind(refLLH(2)), cosd(refLLH(1));
                    -sind(refLLH(2)),                   cosd(refLLH(2)),                    0;
                    -cosd(refLLH(1)) * cosd(refLLH(2)), -cosd(refLLH(1)) * sind(refLLH(2)), -sind(refLLH(1))];

    tarRange = ecef2NED * (pECEF_target - [pECEF_ref(1); pECEF_ref(2); pECEF_ref(3)]);


end

end

== matlab function LOSR/HandleLOSRInput/LOSRGetB2NED ==
  data: roll input; b2NED output; pitch input; hdg input
function b2NED = LOSRGetB2NED(roll, pitch, hdg)
%LOSRGetNED2ECEF Compute transformation matrix from Body to local NED frame
% Input
% roll      : Current aircraft roll angle [deg]
% pitch     : Current aircraft pitch angle [deg]
% heading   : Current aircraft heading angle [deg]
% Output
% b2NED     : Transformation matrix in single 1D array form

% Initialize
b2NED = zeros(1,9);

b2NED(1,1)  = cosd(hdg) * cosd(pitch);
b2NED(1,2)  = -sind(hdg) * cosd(roll) + cosd(hdg) * sind(pitch) * sind(roll);
b2NED(1,3)  = sind(hdg) * sind(roll) + cosd(hdg) * sind(pitch) * cosd(roll);

b2NED(1,4)  = sind(hdg) * cosd(roll);
b2NED(1,5)  = cosd(hdg) * cosd(pitch) + sind(hdg) * sind(pitch) * sind(roll);
b2NED(1,6)  = -cosd(hdg) * sind(roll) + sind(hdg) * sind(pitch) * cosd(roll);

b2NED(1,7)  = -sind(pitch);
b2NED(1,8)  = cosd(pitch) * sind(roll);
b2NED(1,9)  = cosd(pitch) * cosd(roll);

end

== matlab function LOSR/HandleLOSRInput/LOSRGetNED2ECEF ==
  data: lat input; ned2ECEF output; lon input
function ned2ECEF = LOSRGetNED2ECEF(lat, lon)
%LOSRGetNED2ECEF Compute transformation matrix from local NED to ECEF frame
% Input
% lat       : Current aircraft latitude [deg]
% lon       : Current aircraft longitude [deg]
% Output
% ned2ECEF  : Rotation matrix in single 1D array form
% *Note : (ECEF Vecotr) = (ned2ECEF) * (NED Vector) + (ECEF, Reference)

% Initialize
ned2ECEF = zeros(1,9);

% NED to ECEF Transformation Matrix
ned2ECEF(1,1) = -sind(lat)*cosd(lon);
ned2ECEF(1,2) = -sind(lon);
ned2ECEF(1,3) = -cosd(lat)*cosd(lon);

ned2ECEF(1,4) = -sind(lat)*sind(lon);
ned2ECEF(1,5) = cosd(lon);
ned2ECEF(1,6) = -cosd(lat)*sind(lon);

ned2ECEF(1,7) = cosd(lat);
ned2ECEF(1,8) = 0.0;
ned2ECEF(1,9) = -sind(lat);

end
